simulink model "GUIADO"  (R2021b)
settings: Solver=FixedStepAuto  StartTime=0  StopTime=10.0  RelTol=1e-3
settings Model: Creator=verti  LastModifiedBy=verti

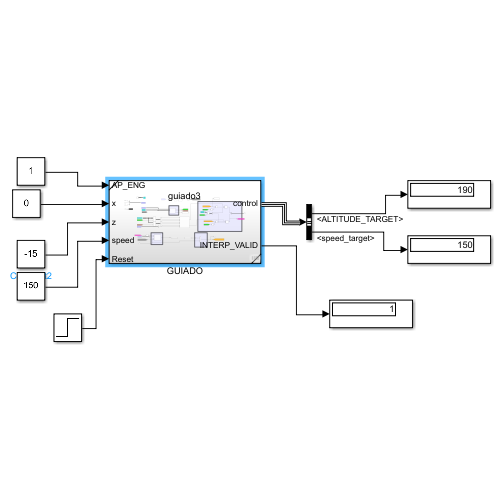
[thumbnail: Simulink's stored preview of the top-level diagram]
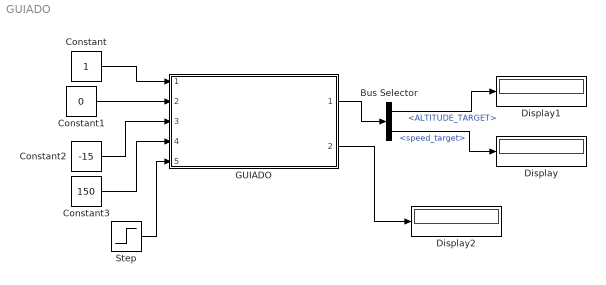
== system GUIADO ==
  Bus Selector : BusSelector  OutputSignals=ALTITUDE_TARGET,speed_target
  Constant : Constant
  Constant1 : Constant  Value=0
  Constant2 : Constant  Value=-15
  Constant3 : Constant  Value=150
  Display : Display
  Display1 : Display
  Display2 : Display
  GUIADO : Subsystem  ReferencedSubsystem=guiado3
  Step : Step  Time=5  SampleTime=0
  wires:
  Constant/1 -> GUIADO/1
  Constant1/1 -> GUIADO/2
  Constant3/1 -> GUIADO/4
  Constant2/1 -> GUIADO/3
  GUIADO/1 -> Bus Selector/1
  Bus Selector/1 -> Display1/1  "<ALTITUDE_TARGET>"
  Bus Selector/2 -> Display/1  "<speed_target>"
  Step/1 -> GUIADO/5
  GUIADO/2 -> Display2/1
